simulink model "AASe"  (R2022b)
settings: Solver=FixedStepDiscrete  StartTime=0.0  StopTime=100  FixedStep=0.01  RelTol=1e-3  EnableMultiTasking=on
libraries: fuzblock x1
settings Model: Creator=marwa  LastModifiedBy=Khaled
settings SolverCC: AlgebraicLoopSolver=TrustRegion  AutoInsertRateTranBlk=on
settings DataIOCC: LimitDataPoints=on
settings OptimizationCC: LifeSpan=inf
settings DebuggingCC: UnconnectedInputMsg=warning  UnconnectedOutputMsg=warning  UnconnectedLineMsg=warning  AllowSymbolicDim=off  SFUnexpectedBacktrackingDiag=warning  SFNoUnconditionalDefaultTransitionDiag=warning  SFExecutionAtInitializationDiag=none  ArithmeticOperatorsInVariantConditions=warning
settings ModelReferenceCC: EnableRefExpFcnMdlSchedulingChecks=on
settings SFSimCC: SimUseLocalCustomCode=off  CustomCodeUndefinedFunction=UseInterfaceOnly
settings RTWCC: RTWUseLocalCustomCode=off  DLArmComputeVersion=19.05
settings CodeAppCC: StateflowObjectComments=on
settings GRTTargetCC: TargetLangStandard=C89/C90 (ANSI)
settings ConfigComp: CovMetricSettings=dw  CovSaveCumulativeToWorkspaceVar=on  CovSaveSingleToWorkspaceVar=on  CovExternalEMLEnable=off  CovSFcnEnable=off

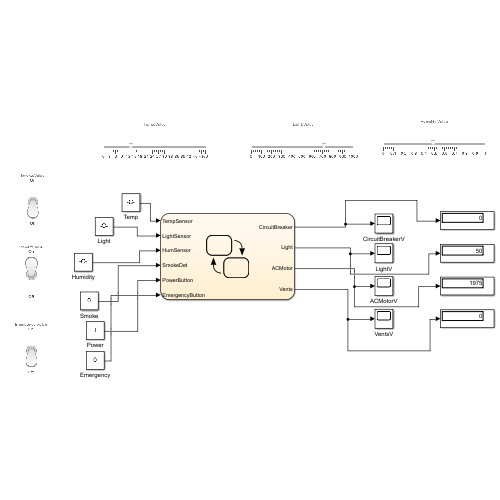
[thumbnail: Simulink's stored preview of the top-level diagram]
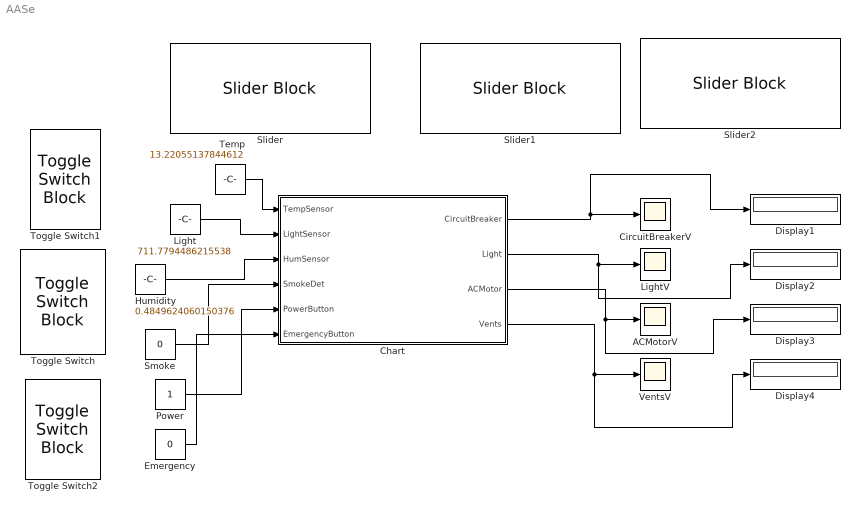
== system AASe ==
  ACMotorV : Scope
  Chart : Stateflow chart  TreatAsAtomicUnit=on
      settings: PortSchema="{\"entries\":[{\"content\":{\"sides\":[{\"content\":{\"connectorIds\":[\"In1\",\"In2\",\"In6\",\"In3\",\"In4\",\"In5\"]},\"type\":\"ConnectorPlacement.EquallySpacedRectSide\",\"uuid\":\"985aadc9-a278-450f-9cf6-a60ed3dedfa6\"},{\"content\":{\"connectorIds\":[\"Out1\",\"Out2\",\"Out3\",\"Out4\"],\"side\":\"RIGHT\"},\"type\":\"ConnectorPlacement.EquallySpacedRectSide\",\"uuid\":\"b5d28c2d-f980-4006-8417-c3abf01696c6\"},{\"content\":{\"connectorIds\":[],\"side\":\"TOP\"},\"type\":\"ConnectorPlacement.EquallySpacedRectSide\",\"uuid\":\"09084e38-e154-4b3b-a97b-f42878e4de9a\"}]},\"type\":\"ConnectorPlacement.EquallySpacedConnector\",\"uuid\":\"fd98585b-3924-471d-992c-1121e6c28ff9\"}],\"packageUris\":[\"http://schema.mathworks.com/mf0/Connector/R2020b\"],\"version\":\"1.0\"}"
  CircuitBreakerV : Scope
  Display{1..4} (4 alike) : Display
  Emergency : Constant  Value=0
  Humidity : Constant  Value=0.4849624060150376
  Light : Constant  Value=711.7794486215538
  LightV : Scope
  Power : Constant
  Slider : SliderBlock  ScaleMax=50
  Slider1 : SliderBlock  ScaleMax=1000
  Slider2 : SliderBlock  ScaleMax=1
  Smoke : Constant  Value=0
  Temp : Constant  Value=13.22055137844612
  Toggle Switch : ToggleSwitchBlock
      settings: Values={{'Off', 'On'}, [0 1]}
  Toggle Switch1 : ToggleSwitchBlock
      settings: Values={{'Off', 'On'}, [0 1]}
  Toggle Switch2 : ToggleSwitchBlock
      settings: Values={{'Off', 'On'}, [0 1]}
  VentsV : Scope
  wires:
  Power/1 -> Chart/4(PowerButton)
  Smoke/1 -> Chart/3(SmokeDet)
  Emergency/1 -> Chart/5(EmergencyButton)
  Temp/1 -> Chart/1(TempSensor)
  Light/1 -> Chart/2(LightSensor)
  Chart/1(CircuitBreaker) -> Display1/1, CircuitBreakerV/1
  Chart/2(Light) -> Display2/1, LightV/1
  Chart/3(ACMotor) -> Display3/1, ACMotorV/1
  Chart/4(Vents) -> Display4/1, VentsV/1
  Humidity/1 -> Chart/6(HumSensor)

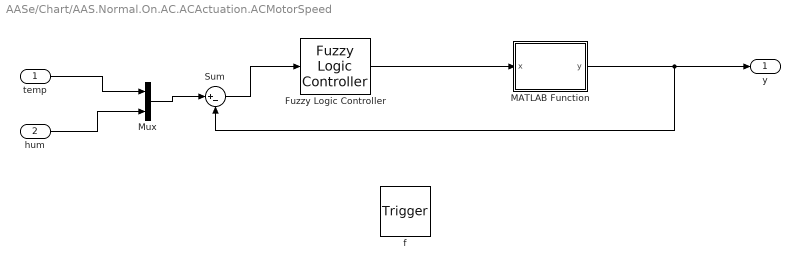
== system AASe/Chart/AAS.Normal.On.AC.ACActuation.ACMotorSpeed ==
  temp : Inport  OutDataTypeStr=double  PortDimensions=1
  hum : Inport  Port=2  OutDataTypeStr=double  PortDimensions=1
  f : TriggerPort  TriggerType=function-call  VariantControl=(inherit)
      settings: CopyFcn=Stateflow.SLINSF.SimulinkMan.removeBlockPreDeleteFcn  PreDeleteFcn=Stateflow.SLINSF.SimulinkMan.unsafePredeleteFcn
  Fuzzy Logic Controller : fuzblock/Fuzzy Logic  Controller  FIS=FuzzyAdvanced  OutputSampleNumber=101  DataType=double  FuzzifiedInputs=off  RuleFiringStrengths=off  RuleOutputs=off  AggregatedOutputs=off  SimulateUsing=Interpreted execution  OutOfRangeInputValueMessage=warning  NoRuleFiredMessage=warning  EmptyOutputFuzzySetMessage=warning
  MATLAB Function : MATLAB Function  TreatAsAtomicUnit=on
  Mux : Mux  Inputs=2
  Sum : Sum  Inputs=|+-
  y : Outport
  wires:
  temp/1 -> Mux/1
  hum/1 -> Mux/2
  MATLAB Function/1(y) -> Sum/2, y/1
  Fuzzy Logic Controller/1 -> MATLAB Function/1(x)
  Sum/1 -> Fuzzy Logic Controller/1
  Mux/1 -> Sum/1

== matlab function AASe/Chart/AAS.Normal.On.AC.ACActuation.ACMotorSpeed/MATLAB Function ==
  data: x input; y output
function y = fcn(x)
y = 1725*x+1725;

== stateflow chart AASe/Chart ==
  state AAS
    state Normal
      entry:
      Vents = 0;
      CircuitBreaker = 0;
      state On
        state Light [parallel]
          settings: executionOrder=2
          state LightSensing [parallel]
            du:
            Illumni = LightSensor;
            settings: executionOrder=1
          state LightActuation [parallel]
            settings: executionOrder=2
            (history)
            state Zero
              entry:
              Light = 0;
              %0 dark
              %1000 light
            state Quarter
              entry:
              Light = 25;
            state Half
              entry:
              Light = 50;
            state Maximum
              entry:
              Light = 100;
            state ThreeQuarter
              entry:
              Light = 75;
            (default) -> Zero
            Quarter -> Half [order 1] : [Illumni < 750]
            Zero -> Quarter : [Illumni < 1000]
            Quarter -> Zero [order 2] : [Illumni >= 1000]
            Half -> Quarter [order 2] : [[Illumni >= 750]]
            ThreeQuarter -> Half [order 2] : [Illumni >= 500]
            Half -> ThreeQuarter [order 1] : [Illumni < 500]
            ThreeQuarter -> Maximum [order 1] : [Illumni < 250]
            Maximum -> ThreeQuarter : [Illumni >= 250]
        state AC [parallel]
          settings: executionOrder=1
          state ACActuation [parallel]
            du:
            ACMotor = ACMotorSpeed(temp,hum)
            settings: executionOrder=3
            state y = ACMotorSpeed(temp,hum) [function]
          state TempSensing [parallel]
            du:
            temp = TempSensor;
            settings: executionOrder=1
          state HumSensing [parallel]
            du:
            hum = HumSensor;
            settings: executionOrder=2
      state Off
        entry:
        Light = 0;
        ACMotor = 0;
        CircuitBreaker = 0;
        Vents = 0;
      (default) -> Off
      Off -> On : [PowerButton == 1]
      On -> Off : [PowerButton == 0]
    state Emergency
      entry:
      Vents = 1;
      CircuitBreaker = 1;
      Light = 100;
      ACMotor = 0;
    (default) -> Normal
    Normal -> Emergency : [EmergencyButton == 1 || SmokeDet == 1]
    Emergency -> Normal : [EmergencyButton == 0 && SmokeDet == 0]
  (default) -> AAS
  data: y function_output; temp function_input double size=1; hum function_input double size=1; CircuitBreaker output; Light output; ACMotor output; Vents output; TempSensor input; LightSensor input; SmokeDet input; PowerButton input; EmergencyButton input; temp local; Illumni local; HumSensor input; hum local
